simulink model "chap1_2"  (Simulink 3.00)
settings: Solver=ode4  StartTime=0.0  StopTime=10  RelTol=1e-3
libraries: simulink3 x1, simulink_extras x1
settings Model: SaveTime=off  SaveOutput=off  Decimation=100

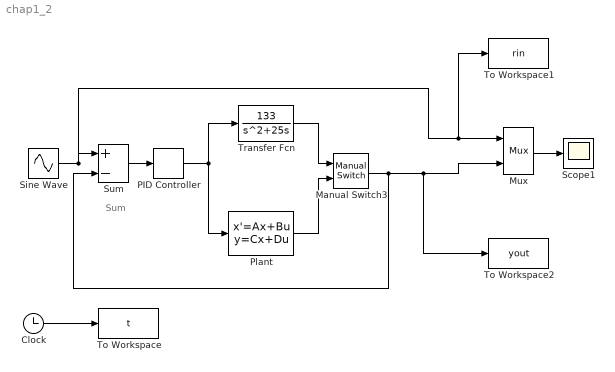
== system chap1_2 ==
  note: Sum
  Clock : Clock
      settings: DisplayTime=off  Decimation=10
  Manual Switch3 : simulink3/Nonlinear/Manual Switch  sw=0  action=0
  Mux : Mux  Inputs=2
      settings: DisplayOption=none
  PID Controller : simulink_extras/Additional Linear/PID Controller  P=60  I=1  D=3
  Plant : StateSpace  A=[0 1;0 -25]  B=[0;133]  C=[1 0]  D=zeros(1)  X0=0
  Scope1 : Scope
      settings: TimeRange=0.2  YMin=-0.051  YMax=-0.041  SaveToWorkspace=off  SaveName=ScopeData  MaxRows=50000  Decimation=0.001  SampleInput=on  SampleTime=0.001
  Sine Wave : Sin  Amplitude=1  Frequency=0.20*2*pi  Phase=0  SampleTime=0
  Sum : Sum  Inputs=|+-  SaturateOnIntegerOverflow=on
  To Workspace : ToWorkspace  VariableName=t  SampleTime=-1  SaveFormat=Matrix
  To Workspace1 : ToWorkspace  VariableName=rin  SampleTime=-1  SaveFormat=Matrix
  To Workspace2 : ToWorkspace  VariableName=yout  SampleTime=-1  SaveFormat=Matrix
  Transfer Fcn : TransferFcn  Numerator=[133]  Denominator=[1 25 0]
  wires:
  Sum/1 -> PID Controller/1
  Sine Wave/1 -> Sum/1, Mux/1, To Workspace1/1
  Mux/1 -> Scope1/1
  Transfer Fcn/1 -> Manual Switch3/1
  Plant/1 -> Manual Switch3/2
  PID Controller/1 -> Transfer Fcn/1, Plant/1
  Clock/1 -> To Workspace/1
  Manual Switch3/1 -> Mux/2, To Workspace2/1, Sum/2
